simulink model "Test3Part3"  (R2024a)
settings: Solver=VariableStepAuto  StartTime=0.0  StopTime=100  RelTol=1e-5
libraries: matrix_library x2
settings Model: Creator=katutu  LastModifiedBy=katutu

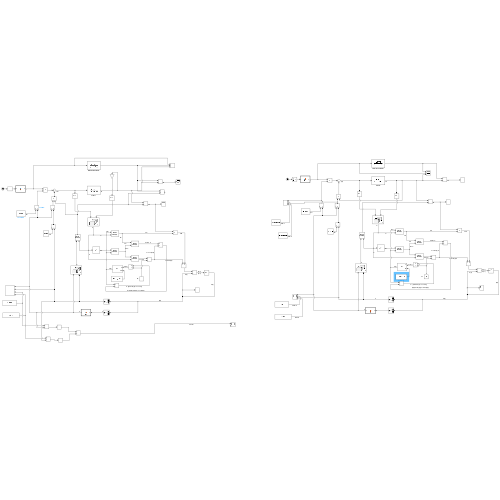
[thumbnail: Simulink's stored preview of the top-level diagram]
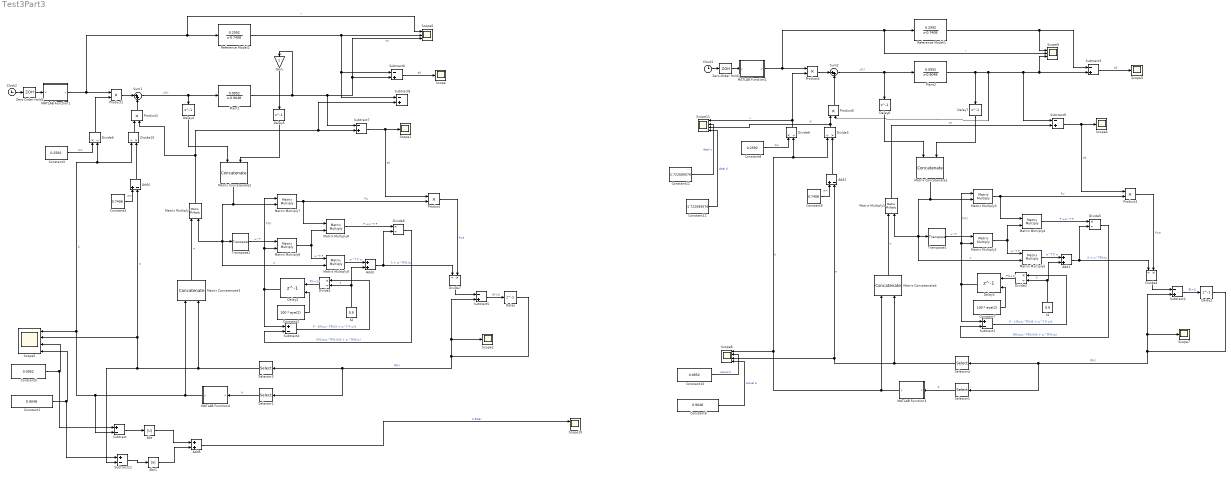
== system Test3Part3 ==
  Abs : Abs  SaturateOnIntegerOverflow=off
  Abs1 : Abs  SaturateOnIntegerOverflow=off
  Add1 : Sum
  Add2 : Sum  Inputs=+-
  Add3 : Sum
  Add4 : Sum  Inputs=+-
  Add5 : Sum
  Clock1 : Clock
  Clock2 : Clock
  Constant1 : Constant  Value=0.9048
  Constant10 : Constant  Value=0.0952
  Constant11 : Constant  Value=2.722689076
  Constant12 : Constant  Value=-1.722689076
  Constant2 : Constant  Value=100 * eye(2)
  Constant3 : Constant  Value=0.2592
  Constant4 : Constant  Value=0.7408
  Constant5 : Constant  Value=0.0952
  Constant6 : Constant  Value=0.9048
  Constant7 : Constant  Value=100 * eye(2)
  Constant8 : Constant  Value=0.2592
  Constant9 : Constant  Value=0.7408
  Delay{,1,4..7} (6 alike) : Delay  DelayLength=1  InitialCondition=0
  Delay2 : Delay  DelayLength=1  InitialConditionSource=Input port  InitialCondition=0
      settings: InputPortMap=u0,p4
  Delay3 : Delay  DelayLength=1  InitialConditionSource=Input port  InitialCondition=0
      settings: InputPortMap=u0,p4
  Divide{1..2,5..6,8..9} (6 alike) : Product  Inputs=*/
  Divide{3..4,7,10} (4 alike) : Product  Inputs=/*
  Gain : Gain
  MATLAB Function1 : MATLAB Function  TreatAsAtomicUnit=on
  MATLAB Function2 : MATLAB Function  TreatAsAtomicUnit=on
  MATLAB Function3 : MATLAB Function  TreatAsAtomicUnit=on
  MATLAB Function4 : MATLAB Function  TreatAsAtomicUnit=on
  Matrix Concatenate1 : Concatenate  Mode=Multidimensional array
  Matrix Concatenate2 : Concatenate  Mode=Multidimensional array
  Matrix Concatenate3 : Concatenate  Mode=Multidimensional array  ConcatenateDimension=2
  Matrix Concatenate4 : Concatenate  Mode=Multidimensional array  ConcatenateDimension=2
  Matrix Multiply{,1..9} (10 alike) : Product  Multiplication=Matrix(*)
  Plant1 : DiscreteTransferFcn  Numerator=[0.0952]  Denominator=[1 -0.9048]
  Plant2 : DiscreteTransferFcn  Numerator=[0.0952]  Denominator=[1 -0.9048]
  Product{,1..5} (6 alike) : Product
  Reference Model1 : DiscreteTransferFcn  Numerator=[0.2592]  Denominator=[1 -0.7408]
  Reference Model2 : DiscreteTransferFcn  Numerator=[0.2592]  Denominator=[1 -0.7408]
  Scope{,1..4,7} (6 alike) : Scope
  Scope10 : Scope  NumInputPorts=2
  Scope11 : Scope  NumInputPorts=4
  Scope5 : Scope  NumInputPorts=4
  Scope6 : Scope  NumInputPorts=3
  Scope8 : Scope  NumInputPorts=4
  Scope9 : Scope  NumInputPorts=3
  Selector1 : Selector  InputPortWidth=2  IndexOptions=Index vector (dialog)  Indices=[1]  OutputSizes=1
  Selector2 : Selector  InputPortWidth=2  IndexOptions=Index vector (dialog)  Indices=[1]  OutputSizes=1
  Selector3 : Selector  InputPortWidth=2  IndexOptions=Index vector (dialog)  Indices=[2]  OutputSizes=1
  Selector4 : Selector  InputPortWidth=2  IndexOptions=Index vector (dialog)  Indices=[2]  OutputSizes=1
  Subtract{,1,4,11} (4 alike) : Sum  Inputs=+-
  Subtract{2..3,5..9} (7 alike) : Sum  Inputs=-+
  Sum1 : Sum  Inputs=|++
  Sum2 : Sum  Inputs=|++
  Transpose1 : matrix_library/Transpose
  Transpose2 : matrix_library/Transpose
  Zero-Order Hold1 : ZeroOrderHold  SampleTime=-1
  Zero-Order Hold2 : ZeroOrderHold  SampleTime=-1
  λ1 : Constant  Value=0.9
  λ2 : Constant  Value=0.9
  wires:
  Matrix Multiply8/1 -> Divide8/1  "P ww^T P"
  Sum1/1 -> Plant1/1, Delay4/1  "u(k)"
  Selector2/1 -> MATLAB Function4/1(u)  "b"
  Divide7/1 -> Subtract5/1
  Matrix Multiply9/1 -> Add3/1  "w^T P w"
  Matrix Concatenate2/1 -> Matrix Multiply7/2, Matrix Multiply/2, Matrix Multiply9/2, Transpose2/1  "w"
  Delay2/1 -> Matrix Multiply6/2, Matrix Multiply7/1, Subtract4/1  "P(k)"
  Divide1/1 -> Delay2/1  "P(k+1)"
  Product1/1 -> Sum1/1
  Constant2/1 -> Delay2/2
  Matrix Multiply6/1 -> Matrix Multiply9/1, Matrix Multiply8/2  "w^T P"
  Plant1/1 -> Subtract7/1, Scope6/3, Subtract6/2, Gain/1  "yp"
  MATLAB Function1/1(y) -> Product1/1, Reference Model2/1, Scope6/1  "r"
  Divide8/1 -> Subtract4/2  "(P(k)ww^TP(k))/(λ + w^TP(k)w)"
  Add3/1 -> Divide7/1, Divide8/2  "λ + w^TP(k)w"
  Divide10/1 -> Product2/1
  Transpose2/1 -> Matrix Multiply6/1  "w^T"
  Selector3/1 -> Subtract11/2, Scope5/2, Add4/2, Matrix Concatenate3/2  "a"
  Subtract4/1 -> Divide1/1  "P - {(Pww^TP)/(λ + w^T P w)}"
  Matrix Multiply7/1 -> Product/2, Matrix Multiply8/1  "Pw"
  λ2/1 -> Add3/2, Divide1/2  "λ"
  MATLAB Function4/1(y) -> Matrix Concatenate3/1, Subtract/2, Divide10/1, Divide9/2, Scope5/1  "b"
  Clock2/1 -> Zero-Order Hold2/1
  Add4/1 -> Divide10/2
  Product2/1 -> Sum1/2
  Product/1 -> Divide7/2  "Pwe"
  Constant3/1 -> Divide9/1  "bm"
  Divide9/1 -> Product1/2
  Zero-Order Hold2/1 -> MATLAB Function1/1(u)
  Constant4/1 -> Add4/1  "am"
  Subtract5/1 -> Delay/1  "θ(+1)"
  Matrix Concatenate3/1 -> Matrix Multiply/1  "w"
  Delay/1 -> Selector3/1, Selector2/1, Scope2/1, Subtract5/2  "θ(k)"
  Constant5/1 -> Subtract/1, Scope5/3
  Constant1/1 -> Subtract11/1, Scope5/4
  Subtract7/1 -> Product/1, Scope1/1  "e0"
  Matrix Multiply/1 -> Product2/2, Subtract7/2, Subtract8/2
  Subtract6/1 -> Scope/1  "e0"
  Gain/1 -> Delay5/1
  Reference Model2/1 -> Subtract6/1, Subtract8/1, Scope6/2
  Delay5/1 -> Matrix Concatenate2/2
  Delay4/1 -> Matrix Concatenate2/1
  Constant7/1 -> Delay3/2
  Product5/1 -> Sum2/2
  Add2/1 -> Divide3/2
  Divide6/1 -> Product4/2, Scope11/1  "c"
  MATLAB Function3/1(y) -> Matrix Concatenate4/1, Divide3/1, Divide6/2, Scope8/1  "b"
  Subtract2/1 -> Delay1/1  "θ(+1)"
  Plant2/1 -> Delay7/1, Product5/2, Subtract9/1, Subtract3/2, Scope9/3  "yp"
  Matrix Multiply4/1 -> Divide5/1  "P ww^T P"
  Sum2/1 -> Delay6/1, Plant2/1  "u(k)"
  Delay1/1 -> Selector4/1, Selector1/1, Scope7/1, Subtract2/2  "θ(k)"
  Delay3/1 -> Matrix Multiply2/2, Matrix Multiply3/1, Subtract1/1  "P(k)"
  Matrix Concatenate4/1 -> Matrix Multiply1/1  "w"
  Matrix Multiply3/1 -> Product3/2, Matrix Multiply4/1  "Pw"
  Divide3/1 -> Scope11/3, Product5/1  "d"
  Zero-Order Hold1/1 -> MATLAB Function2/1(u)
  Subtract3/1 -> Scope3/1  "e0"
  Selector4/1 -> Add2/2, Scope8/3, Matrix Concatenate4/2  "a"
  Reference Model1/1 -> Scope9/1, Subtract3/1
  Clock1/1 -> Zero-Order Hold1/1
  Divide5/1 -> Subtract1/2  "(P(k)ww^TP(k))/(λ + w^TP(k)w)"
  Subtract9/1 -> Product3/1, Scope4/1  "e0"
  λ1/1 -> Add1/2, Divide2/2  "λ"
  Constant9/1 -> Add2/1  "am"
  Constant8/1 -> Divide6/1  "bm"
  Divide2/1 -> Delay3/1  "P(k+1)"
  Subtract1/1 -> Divide2/1  "P - {(Pww^TP)/(λ + w^T P w)}"
  Matrix Multiply2/1 -> Matrix Multiply5/1, Matrix Multiply4/2  "w^T P"
  Add1/1 -> Divide4/1, Divide5/2  "λ + w^TP(k)w"
  Matrix Multiply1/1 -> Subtract9/2
  Product4/1 -> Sum2/1
  Transpose1/1 -> Matrix Multiply2/1  "w^T"
  MATLAB Function2/1(y) -> Product4/1, Scope9/2, Reference Model1/1  "r"
  Selector1/1 -> MATLAB Function3/1(u)  "b"
  Matrix Concatenate1/1 -> Matrix Multiply3/2, Matrix Multiply1/2, Matrix Multiply5/2, Transpose1/1  "w"
  Divide4/1 -> Subtract2/1
  Matrix Multiply5/1 -> Add1/1  "w^T P w"
  Product3/1 -> Divide4/2  "Pwe"
  Delay6/1 -> Matrix Concatenate1/1
  Delay7/1 -> Matrix Concatenate1/2
  Subtract/1 -> Abs/1
  Subtract11/1 -> Abs1/1
  Abs1/1 -> Add5/2
  Abs/1 -> Add5/1
  Add5/1 -> Scope10/1  "2.5star"
  Constant10/1 -> Scope8/2  "actual b"
  Constant6/1 -> Scope8/4  "actual a"
  Constant11/1 -> Scope11/2  "ideal c"
  Constant12/1 -> Scope11/4  "ideal d"

== matlab function Test3Part3/MATLAB Function2 ==
  data: u input; y output
function y = fcn(u)

if(u<50)
    y=1;
else
    y=-1;
end

== matlab function Test3Part3/MATLAB Function3 ==
  data: u input; y output
function y = fcn(u)

e = 0.01;

if(u == 0)
    y = e;

elseif(abs(u) < 0.01)
    y = e * u/abs(u);
else
    y = u;
end

== matlab function Test3Part3/MATLAB Function4 ==
  data: u input; y output
function y = fcn(u)

e = 0.01;

if(u == 0)
    y = e;

elseif(abs(u) < 0.01)
    y = e * u/abs(u);
else
    y = u;
end

== matlab function Test3Part3/MATLAB Function1 ==
  data: u input; y output
function y = fcn(u)

if(u<50)
    y=1;
else
    y=-1;
end
